simulink model "MultirotorPathFollowing"  (R2025b)
settings: Solver=VariableStepAuto  StartTime=0.0  StopTime=5  RelTol=1e-3
libraries: uavalgslib x2, uavutilslib x1
settings Model: Creator=Admin  LastModifiedBy=Admin

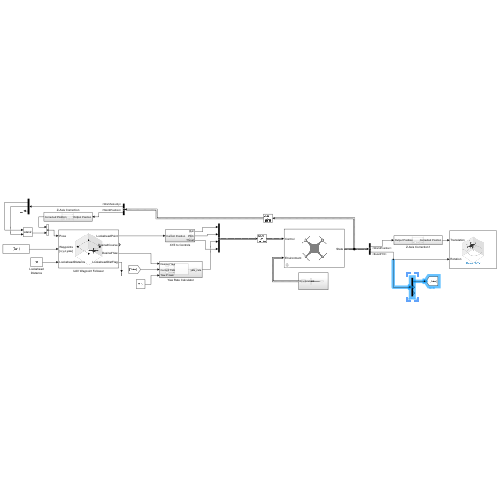
[thumbnail: Simulink's stored preview of the top-level diagram]
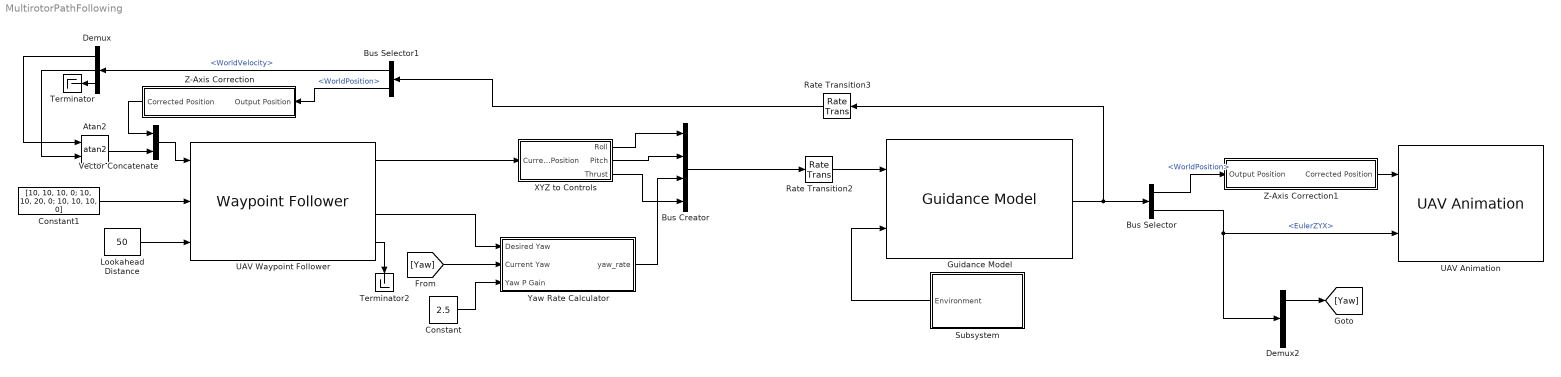
== system MultirotorPathFollowing ==
  Atan2 : Trigonometry  Operator=atan2
  Bus Creator : BusCreator  Inputs=4  OutDataTypeStr=Bus: MultirotorGuidanceControlBus  NonVirtualBus=on
      settings: InheritFromInputs=off
  Bus Selector : BusSelector  OutputSignals=WorldPosition,EulerZYX
  Bus Selector1 : BusSelector  OutputSignals=WorldVelocity,WorldPosition
  Constant : Constant  Value=2.5
  Constant1 : Constant  Value=[10, 10, 10, 0; 10, 10, 20, 0; 10, 10, 10, 0]  OutDataTypeStr=Inherit: Inherit via back propagation
  Demux : Demux  Outputs=3
  Demux2 : Demux  Outputs=3
  Guidance Model : uavalgslib/Guidance Model  ModelType=MultirotorGuidance  NumInstances=1  SpecifiedDataType=double  SimulateUsing=Interpreted execution  InitialWorldPositionMultirotor=[0; 0; 0]  InitialWorldVelocityMultirotor=[0; 0; 0]  InitialEulerZYXMultirotor=[0; 0; 0]  InitialBodyAngularRateRPYMultirotor=[0; 0; 0]  InitialThrustMultirotor=0  InitialNorthFixedWing=0  InitialEastFixedWing=0  InitialHeightFixedWing=0  InitialAirSpeedFixedWing=0  InitialHeadingAngleFixedWing=0  InitialFlightPathAngleFixedWing=0  InitialRollAngleFixedWing=0  InitialRollAngleRateFixedWing=0  PDRollMultirotor=[3402.97,116.67]  PDPitchMultirotor=[3402.97, 116.67]  PYawRateMultirotor=1950  PThrustMultirotor=3900  MassMultirotor=2  PHeightFixedWing=3.9  PHeadingAngleFixedWing=3.9  PFlightPathAngleFixedWing=39  PDRollFixedWing=[3402.97, 116.67]  PAirSpeedFixedWing=1  FlightPathAngleLimitsFixedWing=[-pi/2, pi/2]  StateBusName='MultirotorGuidanceStateBus'  ControlBusName='MultirotorGuidanceControlBus'  EnvironmentBusName='MultirotorGuidanceEnvironmentBus'  DataType=double
  Lookahead Distance : Constant  Value=50
  Rate Transition2 : RateTransition  OutPortSampleTime=0.1
  Rate Transition3 : RateTransition  OutPortSampleTime=0.1
  Subsystem : Subsystem
  Terminator : Terminator
  Terminator2 : Terminator
  UAV Animation : uavutilslib/UAV Animation  NumUAV=1  DynamicUAVConfig=off  UAVType=Multirotor  UAVSize=1  UAVColor=[1 0 0]  UAVTrajectoryAlpha=1  InertialZDirection=Down  RotationFormat=Euler ZYX  DrawMarkers=off  SampleTime=-1
  UAV Waypoint Follower : uavalgslib/Waypoint Follower  UAVType=multirotor  StartFrom=first  TransitionRadiusSource=internal  TransitionRadius=10  MinLookaheadDistance=0.1  HoverAtLastWaypoint=off  YawInput=on  ShowCrossTrackErrorOutput=off  ShowStatusOutput=off  SimulateUsing=Interpreted execution
  Vector Concatenate : Concatenate
  XYZ to Controls : Subsystem
  Yaw Rate Calculator : Subsystem
  Z-Axis Correction : Subsystem
  Z-Axis Correction1 : Subsystem
  wires:
  Subsystem/1(Environment) -> Guidance Model/2
  Rate Transition2/1 -> Guidance Model/1
  Guidance Model/1 -> Rate Transition3/1, Bus Selector/1
  Bus Selector/2 -> Demux2/1, UAV Animation/2  "<EulerZYX>"
  Lookahead Distance/1 -> UAV Waypoint Follower/3
  Rate Transition3/1 -> Bus Selector1/1
  Vector Concatenate/1 -> UAV Waypoint Follower/1
  Bus Selector1/1 -> Demux/1  "<WorldVelocity>"
  Demux/1 -> Atan2/1
  Demux/2 -> Atan2/2
  Atan2/1 -> Vector Concatenate/2
  Demux/3 -> Terminator/1
  UAV Waypoint Follower/4 -> Terminator2/1
  Bus Creator/1 -> Rate Transition2/1
  UAV Waypoint Follower/3 -> Yaw Rate Calculator/1(Desired Yaw)
  Demux2/1 -> [Yaw]
  [Yaw] -> Yaw Rate Calculator/2("Current Yaw ")
  Constant/1 -> Yaw Rate Calculator/3(Yaw P Gain)
  Yaw Rate Calculator/1(yaw_rate) -> Bus Creator/3
  UAV Waypoint Follower/1 -> XYZ to Controls/1(Current Position)
  XYZ to Controls/1(Roll) -> Bus Creator/1
  XYZ to Controls/2(Pitch) -> Bus Creator/2
  XYZ to Controls/3(Thrust) -> Bus Creator/4
  Constant1/1 -> UAV Waypoint Follower/2
  Bus Selector1/2 -> Z-Axis Correction/1(Output Position)  "<WorldPosition>"
  Z-Axis Correction/1(Corrected Position) -> Vector Concatenate/1
  Z-Axis Correction1/1(Corrected Position) -> UAV Animation/1
  Bus Selector/1 -> Z-Axis Correction1/1(Output Position)  "<WorldPosition>"

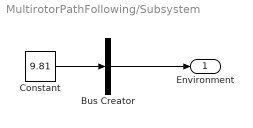
== system MultirotorPathFollowing/Subsystem ==
  Bus Creator : BusCreator  Inputs=1  OutDataTypeStr=Bus: MultirotorGuidanceEnvironmentBus  NonVirtualBus=on
      settings: InheritFromInputs=off
  Constant : Constant  Value=9.81
  Environment : Outport
  wires:
  Bus Creator/1 -> Environment/1
  Constant/1 -> Bus Creator/1

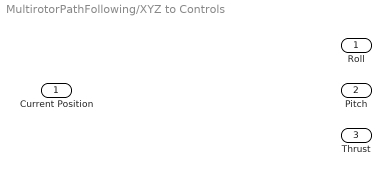
== system MultirotorPathFollowing/XYZ to Controls ==
  Current Position : Inport
  Roll : Outport
  Pitch : Outport  Port=2
  Thrust : Outport  Port=3

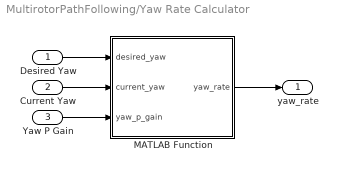
== system MultirotorPathFollowing/Yaw Rate Calculator ==
  Desired Yaw : Inport
  "Current Yaw " : Inport  Port=2
  Yaw P Gain : Inport  Port=3
  MATLAB Function : MATLAB Function  TreatAsAtomicUnit=on
  yaw_rate : Outport
  wires:
  MATLAB Function/1(yaw_rate) -> yaw_rate/1
  Desired Yaw/1 -> MATLAB Function/1(desired_yaw)
  "Current Yaw "/1 -> MATLAB Function/2(current_yaw)
  Yaw P Gain/1 -> MATLAB Function/3(yaw_p_gain)

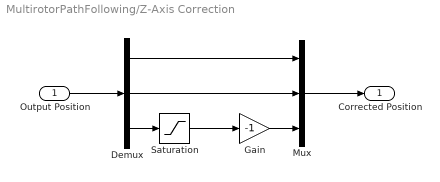
== system MultirotorPathFollowing/Z-Axis Correction ==
  Output Position : Inport
  Demux : Demux  Outputs=3
  Gain : Gain  Gain=-1
  Mux : Mux  Inputs=3
  Saturation : Saturate  UpperLimit=0  LowerLimit=-inf
  Corrected Position : Outport
  wires:
  Mux/1 -> Corrected Position/1
  Output Position/1 -> Demux/1
  Demux/1 -> Mux/1
  Demux/2 -> Mux/2
  Gain/1 -> Mux/3
  Demux/3 -> Saturation/1
  Saturation/1 -> Gain/1

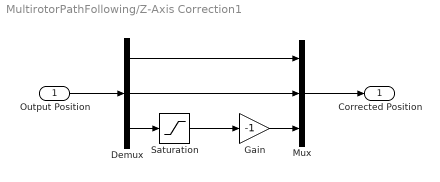
== system MultirotorPathFollowing/Z-Axis Correction1 ==
  Output Position : Inport
  Demux : Demux  Outputs=3
  Gain : Gain  Gain=-1
  Mux : Mux  Inputs=3
  Saturation : Saturate  UpperLimit=0  LowerLimit=-inf
  Corrected Position : Outport
  wires:
  Mux/1 -> Corrected Position/1
  Output Position/1 -> Demux/1
  Demux/1 -> Mux/1
  Demux/2 -> Mux/2
  Gain/1 -> Mux/3
  Demux/3 -> Saturation/1
  Saturation/1 -> Gain/1

== matlab function MultirotorPathFollowing/Yaw Rate Calculator/MATLAB Function ==
  data: desired_yaw input; yaw_rate output; current_yaw input; yaw_p_gain input
function yaw_rate = fcn(desired_yaw, current_yaw, yaw_p_gain)

yaw_rate = yaw_p_gain * wrapToPi(desired_yaw - current_yaw);
